simulink model "espace_etat_2017"  (R2017b)
settings: Solver=VariableStepAuto  StartTime=0.0  StopTime=10.0  RelTol=1e-3
values from neighbouring files (symbols this model uses):
  c_f = 57500    [Vehicule_intelligent.m]
  c_r = 57500    [Vehicule_intelligent.m]
  c_x = 0.35    [Vehicule_intelligent.m]
  c_y = 0.45    [Vehicule_intelligent.m]
  i_eff = 0.3*m    (= 450)    [Vehicule_intelligent.m]
  i_z = 2454    [Vehicule_intelligent.m]
  K = place(A,B1,p)    [Vehicule_intelligent.m]
  l_f = 1.0065    [Vehicule_intelligent.m]
  l_r = 1.4625    [Vehicule_intelligent.m]
  l_w = 40    [Vehicule_intelligent.m]
  m = 1500    [Vehicule_intelligent.m]
  T_r = 0    [Vehicule_intelligent.m]
  v_x = 15    [Vehicule_intelligent.m]
undefined symbols (not defined in the file or in its folder): sigbuilder_block
libraries: simulink x1
settings Model: Creator=szhang6_  LastModifiedBy=bo199
settings SFSimCC: SimUseLocalCustomCode=on
settings RTWCC: RTWUseLocalCustomCode=on

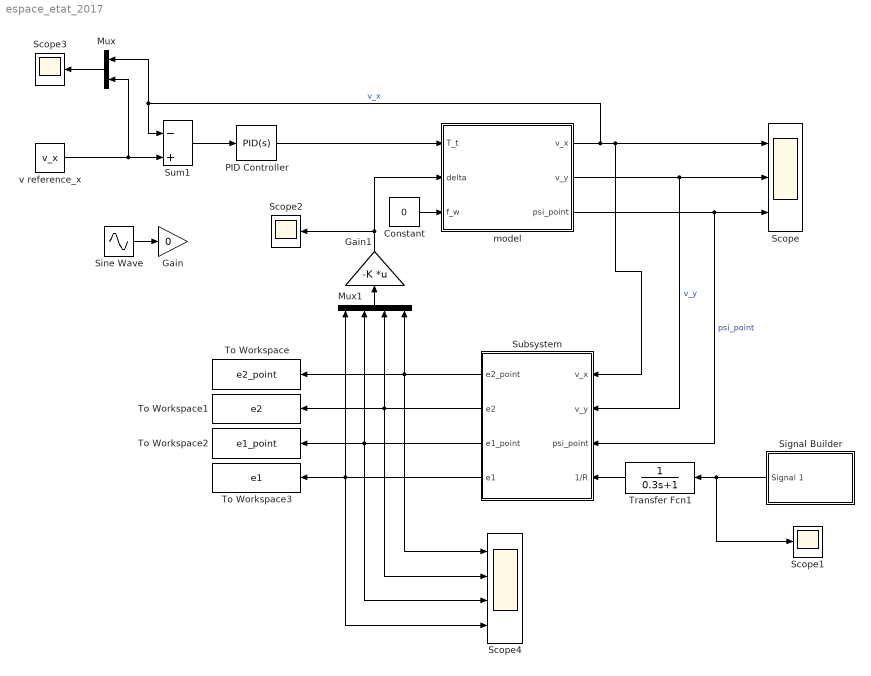
== system espace_etat_2017 ==
  Constant : Constant  Value=0
  Gain : Gain  Gain=0
  Gain1 : Gain  Gain=-K  Multiplication=Matrix(K*u)
  Mux : Mux  Inputs=2
  Mux1 : Mux
  PID Controller : simulink/Continuous/PID Controller  Controller=PID  Form=Parallel  TimeDomain=Continuous-time  SampleTime=-1  IntegratorMethod=Forward Euler  FilterMethod=Forward Euler  ControllerParametersSource=internal  P=250  I=2.8  D=0  UseFilter=on  N=100  TunerSelectOption=Transfer Function Based (PID Tuner App)  InitialConditionSource=internal  InitialConditionForIntegrator=0  InitialConditionForFilter=0  DifferentiatorICPrevScaledInput=0  ExternalReset=none  TrackingMode=off  Kt=1  LimitOutput=off  UpperSaturationLimit=inf  LowerSaturationLimit=-inf  LinearizeAsGain=on  AntiWindupMode=none  Kb=1  POutMin=[]  POutMax=[]  IOutMin=[]  IOutMax=[]  DOutMin=[]  DOutMax=[]  NOutMin=[]  NOutMax=[]  SumOutMin=[]  SumOutMax=[]  SaturationOutMin=[]  SaturationOutMax=[]  PParamMin=[]  PParamMax=[]  IParamMin=[]  IParamMax=[]  DParamMin=[]  DParamMax=[]  NParamMin=[]  NParamMax=[]  KbParamMin=[]  KbParamMax=[]  KtParamMin=[]  KtParamMax=[]  KbOutMin=[]  KbOutMax=[]  KtOutMin=[]  KtOutMax=[]  IntegratorOutMin=[]  IntegratorOutMax=[]  FilterOutMin=[]  FilterOutMax=[]  SumI1OutMin=[]  SumI1OutMax=[]  SumI2OutMin=[]  SumI2OutMax=[]  SumI3OutMin=[]  SumI3OutMax=[]  SumDOutMin=[]  SumDOutMax=[]  DifferentiatorOutMin=[]  DifferentiatorOutMax=[]  FilterDiffOutCoefMin=[]  FilterDiffOutCoefMax=[]  ReciprocalOutMin=[]  ReciprocalOutMax=[]  SumDenOutMin=[]  SumDenOutMax=[]  SumNumOutMin=[]  SumNumOutMax=[]  DivideOutMin=[]  DivideOutMax=[]  IntegratorContinuousStateAttributes=''  IntegratorStateMustResolveToSignalObject=off  IntegratorRTWStateStorageClass=Auto  FilterContinuousStateAttributes=''  FilterStateMustResolveToSignalObject=off  FilterRTWStateStorageClass=Auto  InitialConditionSetting=State (most efficient)
  Scope : Scope  NumInputPorts=3
  Scope1 : Scope
  Scope2 : Scope
  Scope3 : Scope
  Scope4 : Scope  NumInputPorts=4
  Signal Builder : Subsystem  Tag=STV Subsys  LoadFcn=sigbuilder_block('load',[78.75 110.25 1114.5 493.5 ]);  StartFcn=sigbuilder_block('start');  StopFcn=sigbuilder_block('stop');  ClipboardFcn=sigbuilder_block('clipboard');  mask(Sigbuilder block){tuvar=[0:10]}
      mask help: Simulink:masks:SigbuilderBlock_MD
      mask init:
      | if ~strcmp(get_param(bdroot(gcbh),'SimulationStatus'),'stopped') tuvar = sigbuilder_block('maskInit'); end
      settings: CopyFcn=sigbuilder_block('copy');  DeleteFcn=sigbuilder_block('delete');  ModelCloseFcn=sigbuilder_block('modelClose');  PreSaveFcn=sigbuilder_block('preSave');  PauseFcn=sigbuilder_block('pause');  ContinueFcn=sigbuilder_block('continue');  NameChangeFcn=sigbuilder_block('namechange');  OpenFcn=sigbuilder_block('open',[78.75 110.25 1114.5 493.5 ]);  CloseFcn=sigbuilder_block('close');
      mask Display: plot(0, 0, 100, 100,[2, 2, 32, 32, 2], [68, 8, 8, 68, 68],[32, 2], [38, 38], [32, 19, 2],[53, 60, 44], [32, 17, 17, 2],[16, 16, 31, 31]);txt = getActiveGroup(gcbh);text(2, 100, txt,'verticalAlignment', 'top');
  Sine Wave : Sin  Amplitude=0.1  SampleTime=0
  Subsystem : Subsystem
  Sum1 : Sum  Inputs=|-+
  To Workspace : ToWorkspace  VariableName=e2_point  SampleTime=-1
  To Workspace1 : ToWorkspace  VariableName=e2  SampleTime=-1
  To Workspace2 : ToWorkspace  VariableName=e1_point  SampleTime=-1
  To Workspace3 : ToWorkspace  VariableName=e1  SampleTime=-1
  Transfer Fcn1 : TransferFcn  Denominator=[0.3 1]
  model : Subsystem
  "v reference_x " : Constant  Value=v_x
  wires:
  model/1("v_x ") -> Mux/1, Sum1/1, Scope/1, Subsystem/1(v_x)  "v_x"
  model/2("v_y ") -> Subsystem/2(v_y), Scope/2  "v_y"
  Constant/1 -> model/3(f_w)
  Sine Wave/1 -> Gain/1
  PID Controller/1 -> model/1(T_t)
  Mux/1 -> Scope3/1
  "v reference_x "/1 -> Mux/2, Sum1/2
  Sum1/1 -> PID Controller/1
  model/3(psi_point) -> Subsystem/3(psi_point), Scope/3  "psi_point"
  Subsystem/1(e2_point) -> Scope4/1, Mux1/4, To Workspace/1
  Subsystem/3(e1_point) -> Scope4/3, Mux1/2, To Workspace2/1
  Signal Builder/1(Signal 1) -> Scope1/1, Transfer Fcn1/1
  Subsystem/2(e2) -> Scope4/2, Mux1/3, To Workspace1/1
  Subsystem/4(e1) -> Scope4/4, Mux1/1, To Workspace3/1
  Mux1/1 -> Gain1/1
  Gain1/1 -> model/2("delta "), Scope2/1
  Transfer Fcn1/1 -> Subsystem/4(1/R)

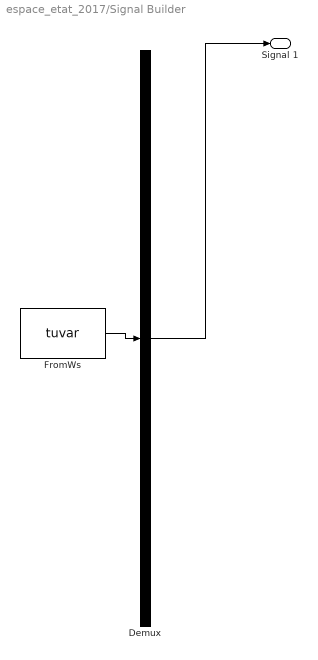
== system espace_etat_2017/Signal Builder ==
  Demux : Demux  Tag=STV Demux  Outputs=1
      settings: DisplayOption=none
  FromWs : FromWorkspace  Tag=STV FromWs  VariableName=tuvar
      SigBuilderData=|
      | common.afterFinalStr = 'Extrapolate'
      | common.sampleTime = 0
      | dataSet.timeRange = [0 10]
      | dataSet.name = 'Group 1'
      | sbobj.Groups.Name = 'Group 1'
      | sbobj.Groups.Signals.Name = 'Signal 1'
      | sbobj.Groups.Signals.XData = [0 2 3 4 5 6 7 8 9 10]
      | sbobj.Groups.Signals.YData = [0 0 0.00333333333333 0.00333333333333 0 1e-05 -0.005 -0.005 0 0]
  Signal 1 : Outport  Tag=STV Outport
  wires:
  Demux/1 -> Signal 1/1
  FromWs/1 -> Demux/1

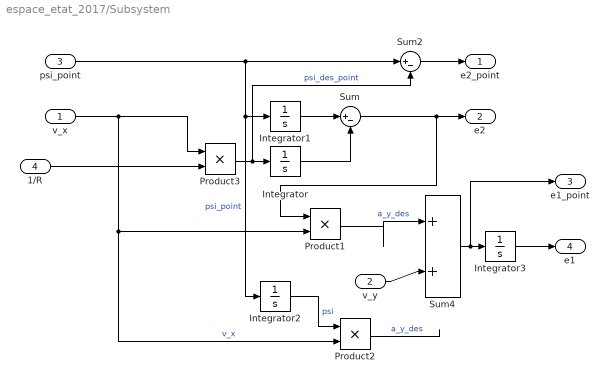
== system espace_etat_2017/Subsystem ==
  v_x : Inport
  v_y : Inport  Port=2
  psi_point : Inport  Port=3
  1/R : Inport  Port=4
  Integrator{,1..3} (4 alike) : Integrator
  Product1 : Product
  Product2 : Product
  Product3 : Product
  Sum : Sum  Inputs=|+-
  Sum2 : Sum  Inputs=|+-
  Sum4 : Sum  Inputs=|++
  e2_point : Outport
  e2 : Outport  Port=2
  e1_point : Outport  Port=3
  e1 : Outport  Port=4
  wires:
  Sum4/1 -> e1_point/1, Integrator3/1
  Product3/1 -> Sum2/2, Integrator/1  "psi_des_point"
  Sum2/1 -> e2_point/1
  Integrator3/1 -> e1/1
  Integrator2/1 -> Product2/1  "psi"
  Integrator1/1 -> Sum/1
  v_x/1 -> Product3/1, Product2/2, Product1/2  "v_x"
  Sum/1 -> Product1/1, e2/1
  Integrator/1 -> Sum/2
  psi_point/1 -> Sum2/1, Integrator2/1, Integrator1/1  "psi_point"
  1/R/1 -> Product3/2
  Product2/1 -> ?  "a_y_des"
  Product1/1 -> Sum4/1  "a_y_des"
  v_y/1 -> Sum4/2

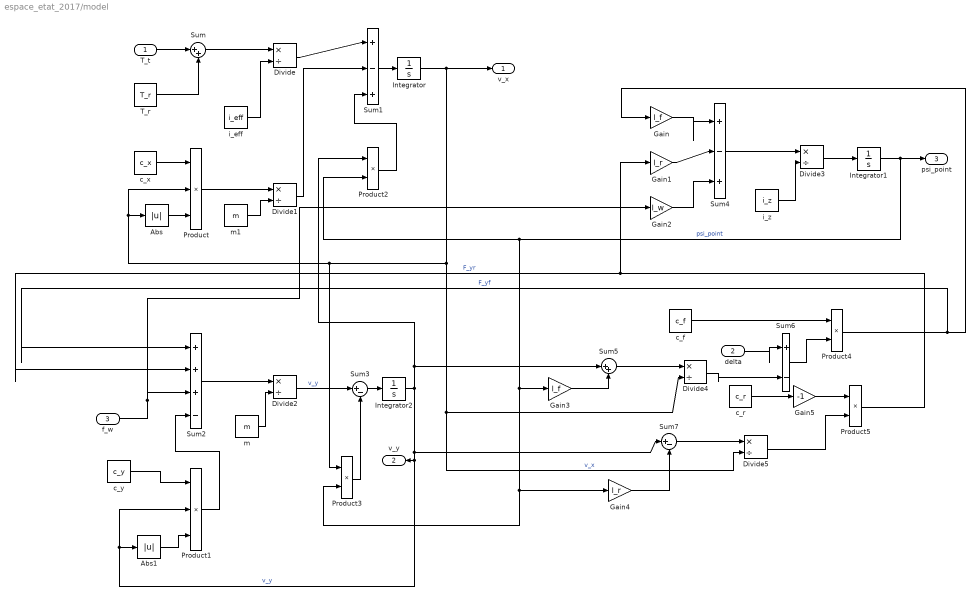
== system espace_etat_2017/model ==
  T_t : Inport
  "delta " : Inport  Port=2
  f_w : Inport  Port=3
  Abs : Abs
  Abs1 : Abs
  Divide{,1..5} (6 alike) : Product  Inputs=*/
  Gain : Gain  Gain=l_f
  Gain1 : Gain  Gain=l_r
  Gain2 : Gain  Gain=l_w
  Gain3 : Gain  Gain=l_f
  Gain4 : Gain  Gain=l_r
  Gain5 : Gain  Gain=-1
  Integrator : Integrator  InitialCondition=10
  Integrator1 : Integrator
  Integrator2 : Integrator  InitialCondition=10
  Product : Product  Inputs=3
  Product1 : Product  Inputs=3
  Product{2..5} (4 alike) : Product
  Sum : Sum  Inputs=|++
  Sum1 : Sum  Inputs=|+-+
  Sum2 : Sum  Inputs=|+++-
  Sum3 : Sum  Inputs=|+-
  Sum4 : Sum  Inputs=|+-+
  Sum5 : Sum  Inputs=|++
  Sum6 : Sum  Inputs=|+-
  Sum7 : Sum  Inputs=|+-
  T_r : Constant  Value=T_r
  c_f : Constant  Value=c_f
  "c_r " : Constant  Value=c_r
  c_x : Constant  Value=c_x
  c_y : Constant  Value=c_y
  i_eff : Constant  Value=i_eff
  i_z : Constant  Value=i_z
  m : Constant  Value=m
  m1 : Constant  Value=m
  "v_x " : Outport
  "v_y " : Outport  Port=2
  psi_point : Outport  Port=3
  wires:
  Gain2/1 -> Sum4/3
  Divide2/1 -> Sum3/1  "v_y"
  Gain1/1 -> Sum4/2
  Product2/1 -> Sum1/3
  c_f/1 -> Product4/1
  Sum2/1 -> Divide2/1
  m/1 -> Divide2/2
  Product3/1 -> Sum3/2
  Sum5/1 -> Divide4/1
  Divide4/1 -> Sum6/2
  Gain3/1 -> Sum5/2
  Product4/1 -> Gain/1, Sum2/1  "F_yf"
  "delta "/1 -> Sum6/1
  T_r/1 -> Sum/2
  T_t/1 -> Sum/1
  Divide3/1 -> Integrator1/1
  Sum6/1 -> Product4/2
  Product1/1 -> Sum2/4
  c_y/1 -> Product1/1
  Abs1/1 -> Product1/3
  Sum/1 -> Divide/1
  Gain/1 -> Sum4/1
  i_eff/1 -> Divide/2
  Divide1/1 -> Sum1/2
  m1/1 -> Divide1/2
  Product/1 -> Divide1/1
  Sum4/1 -> Divide3/1
  i_z/1 -> Divide3/2
  c_x/1 -> Product/1
  Gain4/1 -> Sum7/2
  Sum7/1 -> Divide5/1
  Integrator1/1 -> psi_point/1, Product3/2, Gain4/1, Gain3/1, Product2/2  "psi_point"
  Integrator/1 -> "v_x "/1, Divide5/2, Divide4/2, Product3/1, Abs/1, Product/2  "v_x"
  Divide5/1 -> Product5/2
  Integrator2/1 -> Product1/2, Abs1/1, "v_y "/1, Sum7/1, Product2/1, Sum5/1  "v_y"
  Abs/1 -> Product/3
  Sum1/1 -> Integrator/1
  "c_r "/1 -> Gain5/1
  Divide/1 -> Sum1/1
  Gain5/1 -> Product5/1
  f_w/1 -> Gain2/1, Sum2/3
  Product5/1 -> Sum2/2, Gain1/1  "F_yr"
  Sum3/1 -> Integrator2/1
